simulink model "LAB_05_24_OCT_SIM_KIN_COSDIR"  (R2022b)
settings: Solver=ode4  StartTime=0.0  StopTime=10  FixedStep=0.1  RelTol=1e-3
values from neighbouring files (symbols this model uses):
  I = [Ix 0 0 ... (first row only)    [LAB_03_3_OCT_MAT_EUL_2_VERIFICATION.m]    (also in LAB_03_3_OCT_MAT_EUL_DOUBLESPIN.m = diag([Ix, Iy, Iz]); LAB_03_3_OCT_MAT_EUL_SPINAXIS.m = diag([Ix, Iy, Iz]); LAB_03_3_OCT_MAT_EUL_VECT.m; LAB_04_17_OCT_MAT_KIN.m)
  om_0 = [om_x0, om_y0, om_z0]    [LAB_03_3_OCT_MAT_EUL.m]    (also in LAB_03_3_OCT_MAT_EUL_2_VERIFICATION.m = [om_x0; om_y0; om_z0]; LAB_03_3_OCT_MAT_EUL_DOUBLESPIN.m = [om_x0; om_y0; om_z0]; LAB_03_3_OCT_MAT_EUL_SPINAXIS.m = [om_x0; om_y0; om_z0]; LAB_03_3_OCT_MAT_EUL_VECT.m = [om_x0; om_y0; om_z0])
  phi0 = pi/4    (= 0.785398163397)    [LAB_05_24_OCT_MAT_KIN_COSDIR.m]
  psi0 = pi/4    (= 0.785398163397)    [LAB_05_24_OCT_MAT_KIN_COSDIR.m]
  theta0 = 0    [LAB_02_26_SEPT_MAT_PENDULUM.m]    (also in LAB_05_24_OCT_MAT_KIN_COSDIR.m = 0.785398163397)
libraries: matrix_library x2, sharedutil x2
settings Model: Creator=maria  LastModifiedBy=maria

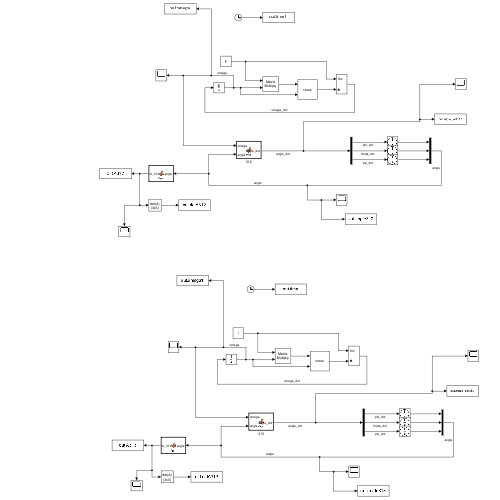
[thumbnail: Simulink's stored preview of the top-level diagram]
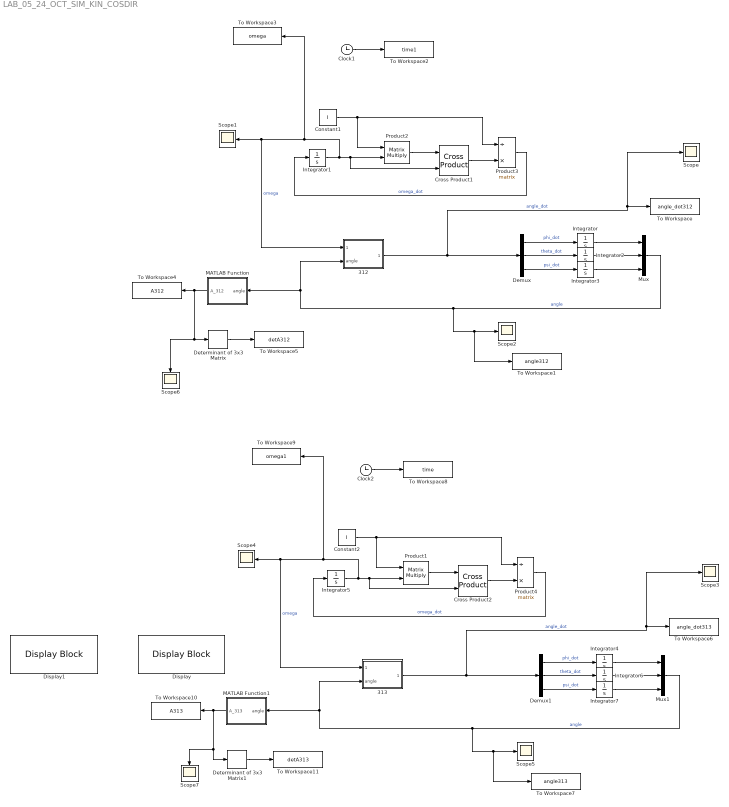
== system LAB_05_24_OCT_SIM_KIN_COSDIR ==
  312 : MATLAB Function  TreatAsAtomicUnit=on
  313 : MATLAB Function  TreatAsAtomicUnit=on
  Clock1 : Clock
  Clock2 : Clock
  Constant1 : Constant  Value=I
  Constant2 : Constant  Value=I
  Cross Product1 : matrix_library/Cross Product
  Cross Product2 : matrix_library/Cross Product
  Demux : Demux  Outputs=3
  Demux1 : Demux  Outputs=3
  Determinant of 3x3 Matrix : sharedutil/Determinant of 3x3 Matrix  aMode=aMode
      settings: LibrarySourceBlock=|
      | aerolibutil/Determinant of
      | 3x3 Matrix
  Determinant of 3x3 Matrix1 : sharedutil/Determinant of 3x3 Matrix  aMode=aMode
      settings: LibrarySourceBlock=|
      | aerolibutil/Determinant of
      | 3x3 Matrix
  Display : DisplayBlock  LabelPosition=Hide  Transparency=1
  Display1 : DisplayBlock  LabelPosition=Hide  Transparency=1
  Integrator : Integrator  InitialCondition=phi0  WrapState=on  WrappedStateUpperValue=2*pi  WrappedStateLowerValue=0
  Integrator1 : Integrator  InitialCondition=om_0
  Integrator2 : Integrator  InitialCondition=theta0  WrapState=on
  Integrator3 : Integrator  InitialCondition=psi0  WrapState=on  WrappedStateUpperValue=2*pi  WrappedStateLowerValue=0
  Integrator4 : Integrator  InitialCondition=phi0  WrapState=on  WrappedStateUpperValue=2*pi  WrappedStateLowerValue=0
  Integrator5 : Integrator  InitialCondition=om_0
  Integrator6 : Integrator  InitialCondition=theta0  WrapState=on
  Integrator7 : Integrator  InitialCondition=psi0  WrapState=on  WrappedStateUpperValue=2*pi  WrappedStateLowerValue=0
  MATLAB Function : MATLAB Function  TreatAsAtomicUnit=on
  MATLAB Function1 : MATLAB Function  TreatAsAtomicUnit=on
  Mux : Mux  Inputs=3
  Mux1 : Mux  Inputs=3
  Product1 : Product  Multiplication=Matrix(*)
  Product2 : Product  Multiplication=Matrix(*)
  Product3 : Product  Inputs=/*  Multiplication=Matrix(*)
  Product4 : Product  Inputs=/*  Multiplication=Matrix(*)
  Scope{,1..7} (8 alike) : Scope
  To Workspace : ToWorkspace  VariableName=angle_dot312  SampleTime=-1
  To Workspace1 : ToWorkspace  VariableName=angle312  SampleTime=-1
  To Workspace10 : ToWorkspace  VariableName=A313  SampleTime=-1
  To Workspace11 : ToWorkspace  VariableName=detA313  SampleTime=-1
  To Workspace2 : ToWorkspace  VariableName=time1  SaveFormat=Timeseries  SampleTime=-1
  To Workspace3 : ToWorkspace  VariableName=omega  SaveFormat=Timeseries  SampleTime=-1
  To Workspace4 : ToWorkspace  VariableName=A312  SampleTime=-1
  To Workspace5 : ToWorkspace  VariableName=detA312  SampleTime=-1
  To Workspace6 : ToWorkspace  VariableName=angle_dot313  SampleTime=-1
  To Workspace7 : ToWorkspace  VariableName=angle313  SampleTime=-1
  To Workspace8 : ToWorkspace  VariableName=time  SaveFormat=Timeseries  SampleTime=-1
  To Workspace9 : ToWorkspace  VariableName=omega1  SaveFormat=Timeseries  SampleTime=-1
  wires:
  Cross Product1/1 -> Product3/2
  Product2/1 -> Cross Product1/1
  Product3/1 -> Integrator1/1  "omega_dot"
  Constant1/1 -> Product3/1, Product2/1
  Integrator1/1 -> Cross Product1/2, Product2/2, 312/1(omega), Scope1/1, To Workspace3/1  "omega"
  Clock1/1 -> To Workspace2/1
  312/1(angle_dot) -> Demux/1, To Workspace/1, Scope/1  "angle_dot"
  Mux/1 -> To Workspace1/1, Scope2/1, 312/2(angle), MATLAB Function/1(angle)  "angle"
  MATLAB Function/1(A_312) -> Determinant of 3x3 Matrix/1, Scope6/1, To Workspace4/1
  Demux/2 -> Integrator2/1  "theta_dot"
  Demux/1 -> Integrator/1  "phi_dot"
  Demux/3 -> Integrator3/1  "psi_dot"
  Integrator2/1 -> Mux/2
  Integrator/1 -> Mux/1
  Integrator3/1 -> Mux/3
  Determinant of 3x3 Matrix/1 -> To Workspace5/1
  Determinant of 3x3 Matrix1/1 -> To Workspace11/1
  Integrator7/1 -> Mux1/3
  Demux1/1 -> Integrator4/1  "phi_dot"
  Mux1/1 -> To Workspace7/1, Scope5/1, 313/2(angle), MATLAB Function1/1(angle)  "angle"
  Integrator6/1 -> Mux1/2
  Demux1/2 -> Integrator6/1  "theta_dot"
  Integrator5/1 -> Cross Product2/2, Product1/2, 313/1(omega), Scope4/1, To Workspace9/1  "omega"
  Product4/1 -> Integrator5/1  "omega_dot"
  Cross Product2/1 -> Product4/2
  Demux1/3 -> Integrator7/1  "psi_dot"
  Product1/1 -> Cross Product2/1
  Clock2/1 -> To Workspace8/1
  313/1(angle_dot) -> Demux1/1, To Workspace6/1, Scope3/1  "angle_dot"
  MATLAB Function1/1(A_313) -> Scope7/1, Determinant of 3x3 Matrix1/1, To Workspace10/1
  Constant2/1 -> Product4/1, Product1/1
  Integrator4/1 -> Mux1/1

== matlab function LAB_05_24_OCT_SIM_KIN_COSDIR/MATLAB Function ==
  data: angle input; A_312 output
function A_312 = fcn(angle)

phi = angle(1);
theta = angle(2);
psi = angle(3);

A_312 = [cos(psi)*cos(phi)-sin(psi)*sin(phi)*sin(theta), cos(psi)*sin(phi)+sin(psi)*cos(phi)*sin(theta), -sin(psi)*cos(theta);
    -sin(phi)*cos(theta), cos(phi)*cos(theta), sin(theta);
    sin(psi)*cos(phi)+cos(psi)*sin(phi)*sin(theta), sin(psi)*sin(phi)-cos(psi)*cos(phi)*sin(theta), cos(theta)*cos(psi)];

end

== matlab function LAB_05_24_OCT_SIM_KIN_COSDIR/312 ==
  data: omega input; angle input; angle_dot output
function angle_dot  = fcn(omega, angle)

om_x = omega(1);
om_y = omega(2);
om_z = omega(3);

phi = angle(1);
theta = angle(2);
psi = angle(3);

phi_dot = (om_z*cos(psi) - om_x*sin(psi))/cos(theta);
theta_dot = om_x*cos(psi) + om_z*sin(psi);
psi_dot = om_y - (om_z*cos(psi) - om_x*sin(psi))*sin(theta)/cos(theta);

angle_dot = [phi_dot; theta_dot; psi_dot];

end

== matlab function LAB_05_24_OCT_SIM_KIN_COSDIR/MATLAB Function1 ==
  data: angle input; A_313 output
function A_313 = fcn(angle)

phi = angle(1);
theta = angle(2);
psi = angle(3);

A_313 = [cos(psi)*cos(phi)-sin(psi)*sin(phi)*cos(theta), cos(psi)*sin(phi)+sin(psi)*cos(phi)*cos(theta), sin(psi)*sin(theta);
    -sin(psi)*cos(phi)-cos(psi)*sin(phi)*cos(theta), -sin(psi)*sin(phi)+cos(psi)*cos(phi)*cos(theta), cos(psi)*sin(theta);
    sin(phi)*sin(theta), -cos(phi)*sin(theta), cos(theta)];

end

== matlab function LAB_05_24_OCT_SIM_KIN_COSDIR/313 ==
  data: omega input; angle input; angle_dot output
function angle_dot  = fcn(omega, angle)

om_x = omega(1);
om_y = omega(2);
om_z = omega(3);

phi = angle(1);
theta = angle(2);
psi = angle(3);

phi_dot = (om_x*sin(psi) + om_y*cos(psi))/sin(theta);
theta_dot = om_x*cos(psi) - om_y*sin(psi);
psi_dot = om_z - (om_x*sin(psi) + om_y*cos(psi))*cos(theta)/sin(theta);

angle_dot = [phi_dot; theta_dot; psi_dot];

end
